simulink library "stopRoutine"  (R2016a)
settings: Solver=ode45  StartTime=0.0  StopTime=10.0  RelTol=1e-3
settings Model: Creator=omaro  LastModifiedBy=oelkawok
settings DataIOCC: LimitDataPoints=on
settings DebuggingCC: AllowSymbolicDim=off

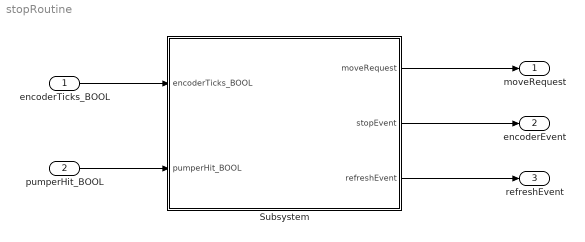
== system stopRoutine ==
  encoderTicks_BOOL : Inport
  pumperHit_BOOL : Inport  Port=2
  Subsystem : Subsystem
  moveRequest : Outport
  encoderEvent : Outport  Port=2
  refreshEvent : Outport  Port=3
  wires:
  encoderTicks_BOOL/1 -> Subsystem/1(encoderTicks_BOOL)
  pumperHit_BOOL/1 -> Subsystem/2(pumperHit_BOOL)
  Subsystem/1(moveRequest) -> moveRequest/1
  Subsystem/2(stopEvent) -> encoderEvent/1
  Subsystem/3(refreshEvent) -> refreshEvent/1

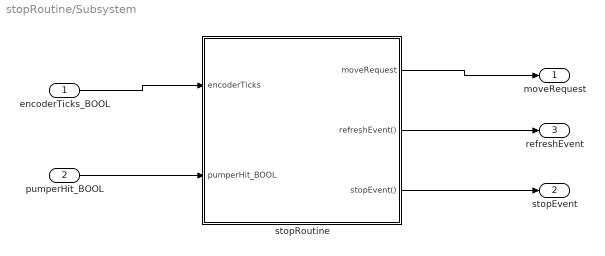
== system stopRoutine/Subsystem ==
  encoderTicks_BOOL : Inport
  pumperHit_BOOL : Inport  Port=2
  stopRoutine : Stateflow chart  TreatAsAtomicUnit=on
  moveRequest : Outport
  stopEvent : Outport  Port=2
  refreshEvent : Outport  Port=3
  wires:
  pumperHit_BOOL/1 -> stopRoutine/2(pumperHit_BOOL)
  encoderTicks_BOOL/1 -> stopRoutine/1(encoderTicks)
  stopRoutine/1(moveRequest) -> moveRequest/1
  stopRoutine/2(refreshEvent()) -> refreshEvent/1
  stopRoutine/3(stopEvent()) -> stopEvent/1

== stateflow chart stopRoutine/Subsystem/stopRoutine ==
  state stopRoutine
    on every(1,tick):
    send(refreshEvent);
    state hitFinish
      en:
      moveRequest = STOP;
      send(stopEvent);
    state Run
    state HitStop
      en:
      moveRequest = STOP;
    state backup
      en:
      moveRequest = BACKWARD;
    (default) -> Run
    hitFinish -> Run : [!pumperHit_BOOL]
    backup -> hitFinish [order 1] : [i>30]
    Run -> HitStop : [pumperHit_BOOL]
    HitStop -> backup : [after(10,tick)]/i = 0;
    backup -> (junction 9) [order 2] : [hasChanged(encoderTicks)]
    (junction 9) -> backup : {i++;}
  (default) -> stopRoutine
  data: encoderTicks input; pumperHit_BOOL input; moveRequest output uint8; i local double; BACKWARD constant double =BACKWARD; STOP constant double =STOP
  events: refreshEvent output FUNCTION_CALL_EVENT; stopEvent output FUNCTION_CALL_EVENT
